simulink model "VanDerPol_T3_C_Simulink"  (R2024b)
settings: Solver=VariableStepAuto  StartTime=0.0  StopTime=30.0  RelTol=1e-3
values from neighbouring files (symbols this model uses):
  a = [1, 5.5, 8.5, 3]    [T1_B_T3_A.m]    (also in T2_B_T3_C.m = 0.5)
  p = [0, 0, 0]    [T1_B_T3_A.m]    (also in T2_A_T3_B.m = [0, 0]; T2_B_T3_C.m = [0, 1])
settings Model: Creator=lukiq  LastModifiedBy=lukiq

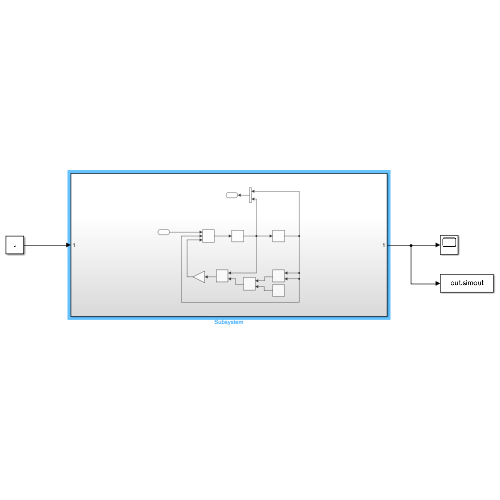
[thumbnail: Simulink's stored preview of the top-level diagram]
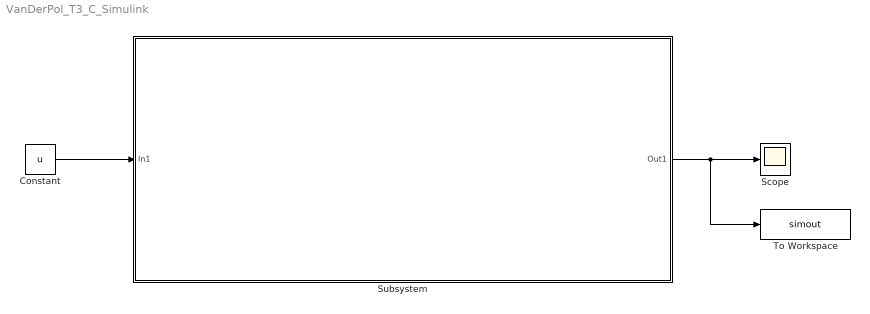
== system VanDerPol_T3_C_Simulink ==
  Constant : Constant  Value=u
  Scope : Scope
  Subsystem : Subsystem
  To Workspace : ToWorkspace  VariableName=simout  SaveFormat=Timeseries  SampleTime=-1
  wires:
  Constant/1 -> Subsystem/1(In1)
  Subsystem/1(Out1) -> To Workspace/1, Scope/1

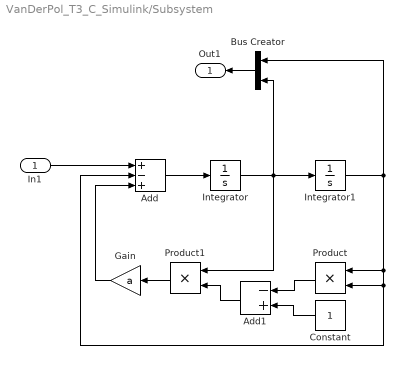
== system VanDerPol_T3_C_Simulink/Subsystem ==
  In1 : Inport
  Add : Sum  Inputs=+-+
  Add1 : Sum  Inputs=-+
  Bus Creator : BusCreator  Inputs=2
  Constant : Constant
  Gain : Gain  Gain=a
  Integrator : Integrator  InitialCondition=p(2)
  Integrator1 : Integrator  InitialCondition=p(1)
  Product : Product
  Product1 : Product
  Out1 : Outport
  wires:
  In1/1 -> Add/1
  Add/1 -> Integrator/1
  Constant/1 -> Add1/2
  Integrator/1 -> Bus Creator/2, Product1/1, Integrator1/1
  Integrator1/1 -> Bus Creator/1, Add/2, Product/2, Product/1
  Product/1 -> Add1/1
  Product1/1 -> Gain/1
  Add1/1 -> Product1/2
  Gain/1 -> Add/3
  Bus Creator/1 -> Out1/1
